simulink model "main"  (R2022b)
settings: Solver=ode4  StartTime=0.0  StopTime=3  FixedStep=0.05  RelTol=1e-3
libraries: MarineRoboticsLib x1
settings Model: Creator=thor  LastModifiedBy=dnad
settings DebuggingCC: UnconnectedInputMsg=warning  UnconnectedOutputMsg=warning  UnconnectedLineMsg=warning
settings ModelReferenceCC: EnableRefExpFcnMdlSchedulingChecks=on
settings RTWCC: DLArmComputeVersion=19.05

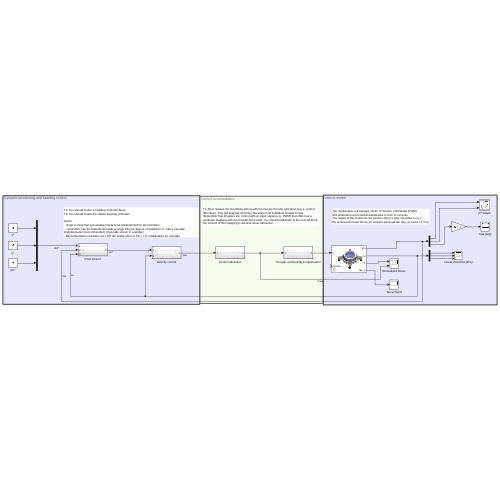
[thumbnail: Simulink's stored preview of the top-level diagram]
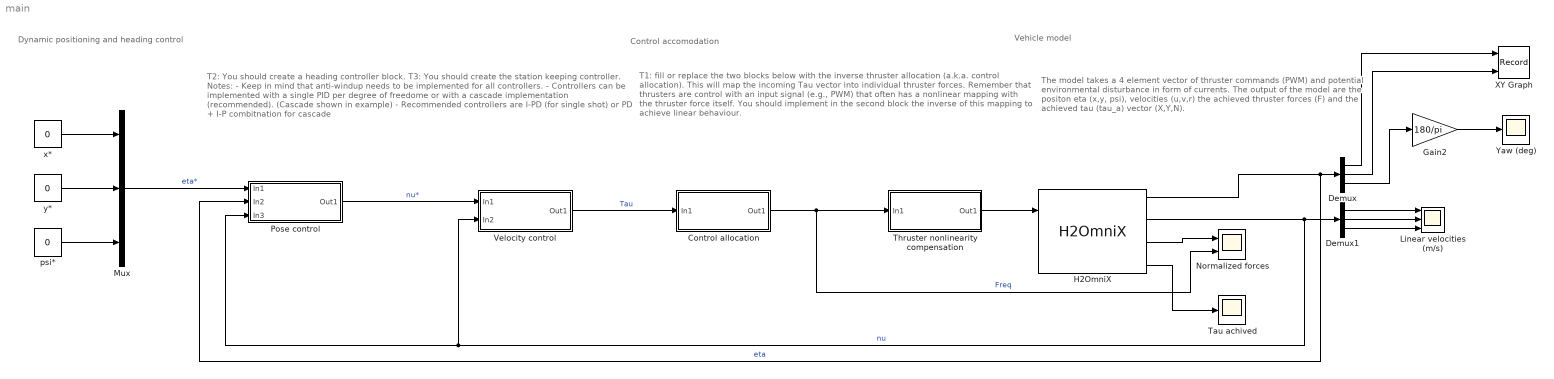
== system main ==
  note: T2: You should create a heading controller block.
      | T3: You should create the station keeping controller.
      |
      | Notes:
      |  - Keep in mind that anti-windup needs to be implemented for all controllers.
      |  - Controllers can be implemented with a single PID per degree of freedome or  with a cascade implementation (recommended). (Cascade shown in example)
      | - Recommended controllers are I-PD (for single shot) or PD + I-P combitnation for cascade
  note: Dynamic positioning and heading control
  note: T1: fill or replace the two blocks below with the inverse thruster allocation (a.k.a. control allocation). This will map the incoming Tau vector into individual thruster forces. Remember that thrusters are control with an input signal (e.g., PWM) that often has a nonlinear mapping with the thruster force itself. You should implement in the second block the inverse of this mapping to achieve linear behaviour.
  note: Vehicle model
  note: Control accomodation
  note: The model takes a 4 element vector of thruster commands (PWM)
      | and potential environmental disturbance in form of currents.
      | The output of the model are the positon eta (x,y, psi), velocities (u,v,r)
      | the achieved thruster forces (F) and the achieved tau (tau_a) vector (X,Y,N).
  Control allocation : Subsystem
  Demux : Demux  Outputs=3
  Demux1 : Demux  Outputs=3
  Gain2 : Gain  Gain=180/pi
  H2OmniX : MarineRoboticsLib/H2OmniX  alpha=[2.1,2.1,0.4]  beta=[1,1,0.24]  betaa=[0,0,0]  nu0=[0,0,0]  eta0=[0,0,0]
  Linear velocities (m/s) : Scope  NumInputPorts=3
  Mux : Mux  Inputs=3
  Normalized forces : Scope  NumInputPorts=2
  Pose control : Subsystem
  Tau achived : Scope
  Thruster nonlinearity compensation : Subsystem
  Velocity control : Subsystem
  XY Graph : Record  FileSettingsInternal="{\"entries\":[{\"content\":{\"excelSettings\":{\"content\":{},\"type\":\"Streamout.ExcelSettings\"}},\"type\":\"Streamout.FileSettingStorage\",\"uuid\":\"ec748efd-57ad-47e0-85f9-0baefcb39d31\"}],\"packageUris\":[\"http://schema.mathworks.com/mf0/streamout_blocks/R2020a\"],\"version\":\"1.0\"}"  Layout=[1 1]  SignalsInternal="{\"entries\":[{\"content\":{\"signals\":[{\"content\":{\"blockPath\":[\"main/XY Graph\"],\"channel\":[],\"dimensions\":[1],\"domain\":\"main/XY Graph\",\"lineColor\":\"#a2142f\",\"plots\":[1],\"port\":1,\"sid\":[],\"signalID\":3213,\"signalName\":\"XY Graph:1\"},\"type\":\"RecordBlkView.Signal\",\"uuid\":\"1619c62f-cd73-4bad-8cdb-f255ae39850c\"},{\"content\":{\"blockPath\":[\"main/XY Graph\"],\"channel\":[],\"dimensions\":[1],\"domain\":\"main/XY Graph\",\"lineColor\":\"#139fff\",\"plots\":[1],\"port\":2,\"sid\":[],\"signalID\":3216,\"signalName\":\"XY Graph:2\"},\"type\":\"RecordBlkView.Signal\",\"uuid\":\"bcfb5777-8d5a-4213-8187-4a0b2d40aaeb\"}]},\"type\":\"RecordBlkView.InputSignals\",\"uuid\":\"524c4619-0f0c-4556-b67b-dcc7924ed330\"}],\"packageUris\":[\"http://schema.mathworks.com/mf0/streamout_blocks/R2020a\"],\"version\":\"1.0\"}"  VisualizationBindings="{\"xyplotplugin\":{\"info\":[{\"series\":[{\"bindingParametersList\":[{\"parameter\":\"X-Axis\",\"signalID\":3213,\"signalName\":\"XY Graph:1\"},{\"parameter\":\"Y-Axis\",\"signalID\":3216,\"signalName\":\"XY Graph:2\"}],\"seriesID\":11415}],\"subplotID\":1}]}}"  CompatibilityTag=XY
  Yaw (deg) : Scope
  psi* : Constant  Value=0
  x* : Constant  Value=0
  y* : Constant  Value=0
  wires:
  H2OmniX/1 -> Demux/1, Pose control/2(In2)  "eta"
  Demux/1 -> XY Graph/1
  Demux/2 -> XY Graph/2
  H2OmniX/2 -> Pose control/3(In3), Velocity control/2(In2), Demux1/1  "nu"
  Demux1/1 -> Linear velocities (m/s)/1
  Demux1/2 -> Linear velocities (m/s)/2
  Demux1/3 -> Linear velocities (m/s)/3
  Demux/3 -> Gain2/1
  Gain2/1 -> Yaw (deg)/1
  H2OmniX/3 -> Normalized forces/1
  H2OmniX/4 -> Tau achived/1
  Control allocation/1(Out1) -> Thruster nonlinearity compensation/1(In1), Normalized forces/2  "Freq"
  Thruster nonlinearity compensation/1(Out1) -> H2OmniX/1
  Velocity control/1(Out1) -> Control allocation/1(In1)  "Tau"
  Pose control/1(Out1) -> Velocity control/1(In1)  "nu*"
  Mux/1 -> Pose control/1(In1)  "eta*"
  x*/1 -> Mux/1
  y*/1 -> Mux/2
  psi*/1 -> Mux/3

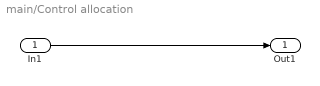
== system main/Control allocation ==
  In1 : Inport
  Out1 : Outport
  wires:
  In1/1 -> Out1/1

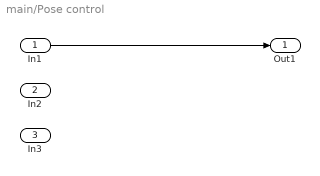
== system main/Pose control ==
  In1 : Inport
  In2 : Inport  Port=2
  In3 : Inport  Port=3
  Out1 : Outport
  wires:
  In1/1 -> Out1/1

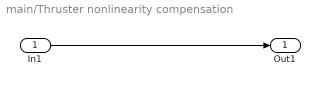
== system main/Thruster nonlinearity compensation ==
  In1 : Inport
  Out1 : Outport
  wires:
  In1/1 -> Out1/1

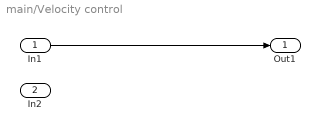
== system main/Velocity control ==
  In1 : Inport
  In2 : Inport  Port=2
  Out1 : Outport
  wires:
  In1/1 -> Out1/1
